simulink model "zad2"  (R2017a)
settings: Solver=VariableStepAuto  StartTime=0.0  StopTime=10.0  RelTol=1e-3
settings Model: Creator=DoktorHax  LastModifiedBy=DoktorHax

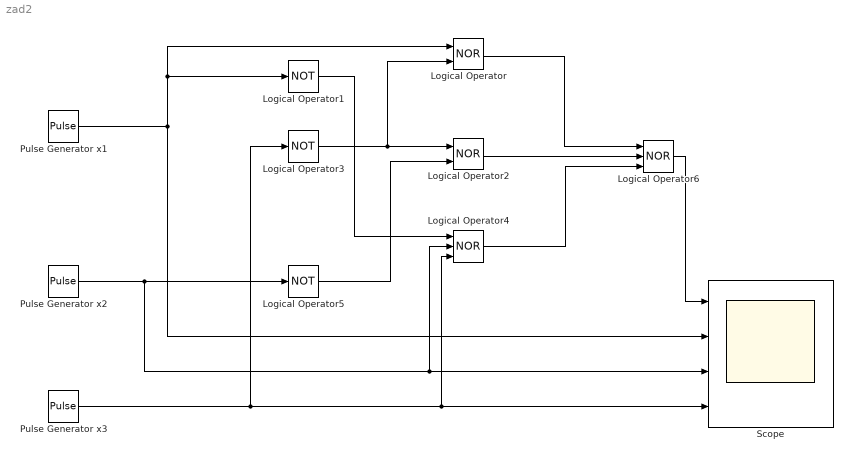
== system zad2 ==
  Logical Operator : Logic  Operator=NOR  AllPortsSameDT=off  OutDataTypeStr=boolean
  Logical Operator1 : Logic  Operator=NOT  AllPortsSameDT=off  OutDataTypeStr=boolean
  Logical Operator2 : Logic  Operator=NOR  AllPortsSameDT=off  OutDataTypeStr=boolean
  Logical Operator3 : Logic  Operator=NOT  AllPortsSameDT=off  OutDataTypeStr=boolean
  Logical Operator4 : Logic  Operator=NOR  Inputs=3  AllPortsSameDT=off  OutDataTypeStr=boolean
  Logical Operator5 : Logic  Operator=NOT  AllPortsSameDT=off  OutDataTypeStr=boolean
  Logical Operator6 : Logic  Operator=NOR  Inputs=3  AllPortsSameDT=off  OutDataTypeStr=boolean
  Pulse Generator x1 : DiscretePulseGenerator  PulseType=Time based  PulseWidth=50
  Pulse Generator x2 : DiscretePulseGenerator  PulseType=Time based  Period=4  PulseWidth=50
  Pulse Generator x3 : DiscretePulseGenerator  PulseType=Time based  Period=8  PulseWidth=50
  Scope : Scope  NumInputPorts=4
  wires:
  Logical Operator/1 -> Logical Operator6/1
  Logical Operator2/1 -> Logical Operator6/2
  Pulse Generator x2/1 -> Logical Operator4/2, Scope/3, Logical Operator5/1
  Logical Operator6/1 -> Scope/1
  Pulse Generator x1/1 -> Logical Operator1/1, Logical Operator/1, Scope/2
  Pulse Generator x3/1 -> Logical Operator3/1, Logical Operator4/3, Scope/4
  Logical Operator4/1 -> Logical Operator6/3
  Logical Operator3/1 -> Logical Operator2/1, Logical Operator/2
  Logical Operator1/1 -> Logical Operator4/1
  Logical Operator5/1 -> Logical Operator2/2
